simulink model "Example_8_4c"  (R2014a)
settings: Solver=ode45  StartTime=0.0  StopTime=10.0  RelTol=1e-3
libraries: simulink x8, dsparch4 x1
settings Model: Creator=Lee Edwards  LastModifiedBy=Lee
settings DataIOCC: SignalLoggingSaveFormat=ModelDataLogs
settings OptimizationCC: ExpressionDepthLimit=2147483647
settings DebuggingCC: UnderspecifiedInitializationDetection=Classic  FcnCallInpInsideContextMsg=UseLocalSettings  StateNameClashWarn=warning  StrictBusMsg=Warning
settings GRTTargetCC: CombineOutputUpdateFcns=off  GRTInterface=on

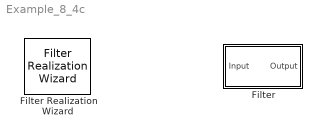
== system Example_8_4c ==
  Filter : Subsystem  Tag=FilterWizardSubSystem
      settings: ErrorFcn=dspFilterRealizedInBasicElemsAlgLoopErrFcnCallback
  Filter Realization Wizard : dsparch4/Filter Realization Wizard

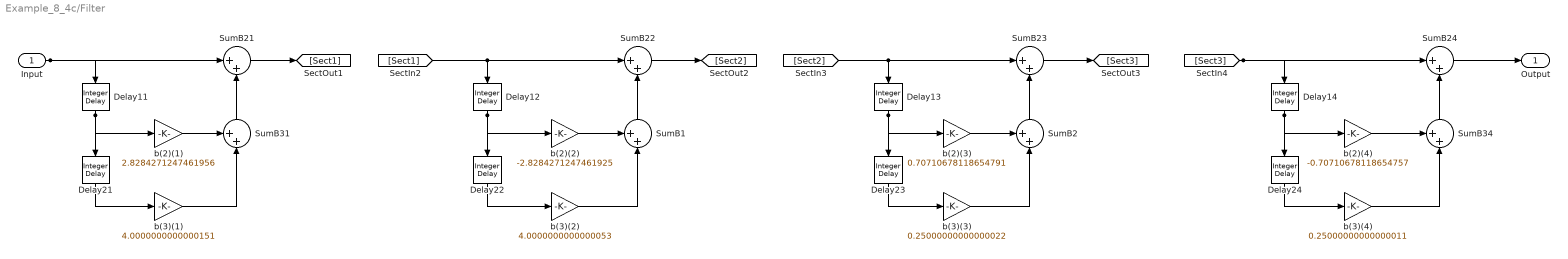
== system Example_8_4c/Filter ==
  Input : Inport
  Delay{11..14,21..24} (8 alike) : simulink/Discrete/Integer Delay  NumDelays=1  vinit=0.0  samptime=-1
  SumB{1..2,31,34} (4 alike) : Sum  Inputs=++|  RndMeth=Nearest  SaturateOnIntegerOverflow=on  OutDataTypeStr=Inherit: Same as first input
  SumB{21..24} (4 alike) : Sum  Inputs=|++  RndMeth=Nearest  SaturateOnIntegerOverflow=on  OutDataTypeStr=Inherit: Same as first input
  b(2)(1) : Gain  Gain=2.8284271247461956  ParamDataTypeStr=float('double')  RndMeth=Nearest  SaturateOnIntegerOverflow=on  OutDataTypeStr=Inherit: Same as input
  b(2)(2) : Gain  Gain=-2.8284271247461925  ParamDataTypeStr=float('double')  RndMeth=Nearest  SaturateOnIntegerOverflow=on  OutDataTypeStr=Inherit: Same as input
  b(2)(3) : Gain  Gain=0.70710678118654791  ParamDataTypeStr=float('double')  RndMeth=Nearest  SaturateOnIntegerOverflow=on  OutDataTypeStr=Inherit: Same as input
  b(2)(4) : Gain  Gain=-0.70710678118654757  ParamDataTypeStr=float('double')  RndMeth=Nearest  SaturateOnIntegerOverflow=on  OutDataTypeStr=Inherit: Same as input
  b(3)(1) : Gain  Gain=4.0000000000000151  ParamDataTypeStr=float('double')  RndMeth=Nearest  SaturateOnIntegerOverflow=on  OutDataTypeStr=Inherit: Same as input
  b(3)(2) : Gain  Gain=4.0000000000000053  ParamDataTypeStr=float('double')  RndMeth=Nearest  SaturateOnIntegerOverflow=on  OutDataTypeStr=Inherit: Same as input
  b(3)(3) : Gain  Gain=0.25000000000000022  ParamDataTypeStr=float('double')  RndMeth=Nearest  SaturateOnIntegerOverflow=on  OutDataTypeStr=Inherit: Same as input
  b(3)(4) : Gain  Gain=0.25000000000000011  ParamDataTypeStr=float('double')  RndMeth=Nearest  SaturateOnIntegerOverflow=on  OutDataTypeStr=Inherit: Same as input
  Output : Outport
  wires:
  Input/1 -> SumB21/1, Delay11/1
  Delay11/1 -> b(2)(1)/1, Delay21/1
  Delay21/1 -> b(3)(1)/1
  b(3)(1)/1 -> SumB31/2
  b(2)(1)/1 -> SumB31/1
  SumB31/1 -> SumB21/2
  SumB21/1 -> [Sect1]
  [Sect1] -> SumB22/1, Delay12/1
  Delay12/1 -> b(2)(2)/1, Delay22/1
  Delay22/1 -> b(3)(2)/1
  b(2)(2)/1 -> SumB1/1
  SumB1/1 -> SumB22/2
  SumB22/1 -> [Sect2]
  b(3)(2)/1 -> SumB1/2
  [Sect2] -> SumB23/1, Delay13/1
  Delay13/1 -> b(2)(3)/1, Delay23/1
  Delay23/1 -> b(3)(3)/1
  b(2)(3)/1 -> SumB2/1
  b(3)(3)/1 -> SumB2/2
  SumB2/1 -> SumB23/2
  SumB23/1 -> [Sect3]
  [Sect3] -> SumB24/1, Delay14/1
  Delay14/1 -> b(2)(4)/1, Delay24/1
  Delay24/1 -> b(3)(4)/1
  b(2)(4)/1 -> SumB34/1
  SumB34/1 -> SumB24/2
  b(3)(4)/1 -> SumB34/2
  SumB24/1 -> Output/1
